simulink library "csc_cgs_coast_guidance_system_lib"  (R2015b)
settings: Solver=ode45  StartTime=0.0  StopTime=10.0  RelTol=1e-3
libraries: util_info_lib x1, util_common_lib x1, csu_arg_aimpoint_roll_guidance_lib x1
settings Model: Creator=Nilesh  LastModifiedBy=Mark Agbayani
settings DataIOCC: SaveFormat=Array
settings DebuggingCC: UnderspecifiedInitializationDetection=Classic  MergeDetectMultiDrivingBlocksExec=none  SolverPrmCheckMsg=warning  StateNameClashWarn=warning
settings HardwareCC: ProdBitPerPointer=32  ProdLargestAtomicFloat=None  ProdIntDivRoundTo=Undefined  ProdEndianess=Unspecified  ProdWordSize=32  ProdHWDeviceType=32-bit Generic
settings GRTTargetCC: GeneratePreprocessorConditionals=Disable all
settings ConfigComp: CovModelRefEnable=Off  CovSFcnEnable=off

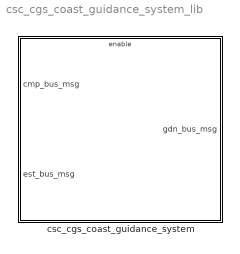
== system csc_cgs_coast_guidance_system_lib ==
  csc_cgs_coast_guidance_system : Subsystem

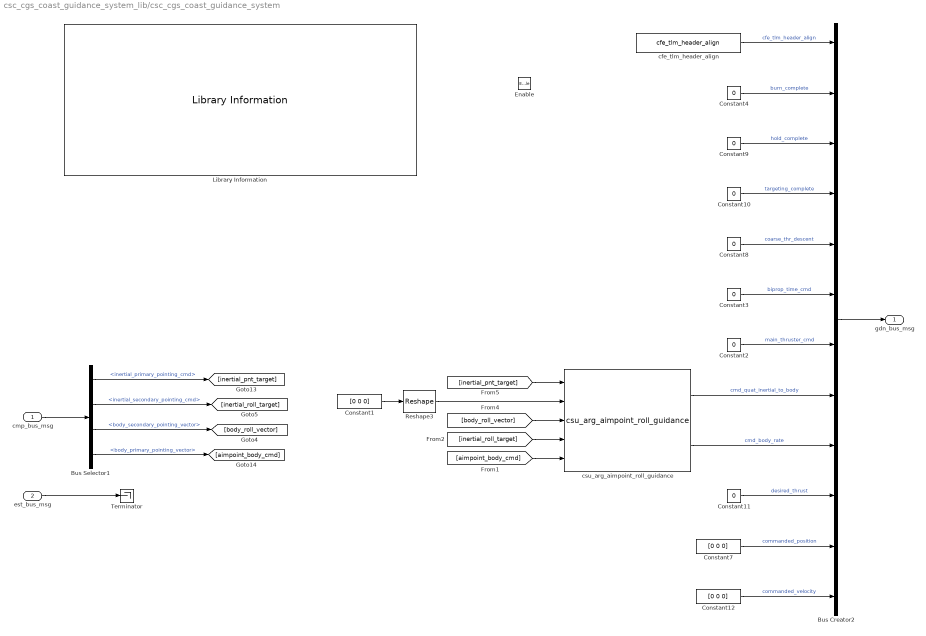
== system csc_cgs_coast_guidance_system_lib/csc_cgs_coast_guidance_system ==
  cmp_bus_msg : Inport
  est_bus_msg : Inport  Port=2
  Enable : EnablePort
  Bus Selector1 : BusSelector  OutputSignals=inertial_primary_pointing_cmd,inertial_secondary_pointing_cmd,body_secondary_pointing_vector,body_primary_pointing_vector
  Bus Creator2 : BusCreator  Inputs=12  OutDataTypeStr=Bus: gdn_bus_msg  NonVirtualBus=on
  Constant1 : Constant  Value=[0 0 0]
  Constant{3..4,8..10} (5 alike) : Constant  Value=0  OutDataTypeStr=uint8
  Constant11 : Constant  Value=0
  Constant12 : Constant  Value=[0 0 0]
  Constant2 : Constant  Value=0
  Constant7 : Constant  Value=[0 0 0]
  Library Information : util_info_lib/Library Information  owner='jkaidy'
  Reshape3 : Reshape  OutputDimensionality=Column vector (2-D)
  Terminator : Terminator
  cfe_tlm_header_align : util_common_lib/cfe_tlm_header_align
  csu_arg_aimpoint_roll_guidance : csu_arg_aimpoint_roll_guidance_lib/csu_arg_aimpoint_roll_guidance
  gdn_bus_msg : Outport  OutDataTypeStr=Bus: gdn_bus_msg
  wires:
  Constant4/1 -> Bus Creator2/2  "burn_complete"
  Constant7/1 -> Bus Creator2/11  "commanded_position"
  Constant12/1 -> Bus Creator2/12  "commanded_velocity"
  Constant3/1 -> Bus Creator2/6  "biprop_time_cmd"
  cfe_tlm_header_align/1 -> Bus Creator2/1  "cfe_tlm_header_align"
  Constant10/1 -> Bus Creator2/4  "targeting_complete"
  Constant9/1 -> Bus Creator2/3  "hold_complete"
  csu_arg_aimpoint_roll_guidance/2 -> Bus Creator2/9  "cmd_body_rate"
  csu_arg_aimpoint_roll_guidance/1 -> Bus Creator2/8  "cmd_quat_inertial_to_body"
  Bus Creator2/1 -> gdn_bus_msg/1
  Constant2/1 -> Bus Creator2/7  "main_thruster_cmd"
  Constant8/1 -> Bus Creator2/5  "coarse_thr_descent"
  Constant11/1 -> Bus Creator2/10  "desired_thrust"
  cmp_bus_msg/1 -> Bus Selector1/1
  Bus Selector1/3 -> [body_roll_vector]  "<body_secondary_pointing_vector>"
  Bus Selector1/2 -> [inertial_roll_target]  "<inertial_secondary_pointing_cmd>"
  Bus Selector1/1 -> [inertial_pnt_target]  "<inertial_primary_pointing_cmd>"
  est_bus_msg/1 -> Terminator/1
  Constant1/1 -> Reshape3/1
  [body_roll_vector] -> csu_arg_aimpoint_roll_guidance/3
  [inertial_roll_target] -> csu_arg_aimpoint_roll_guidance/4
  Reshape3/1 -> csu_arg_aimpoint_roll_guidance/2
  [inertial_pnt_target] -> csu_arg_aimpoint_roll_guidance/1
  Bus Selector1/4 -> [aimpoint_body_cmd]  "<body_primary_pointing_vector>"
  [aimpoint_body_cmd] -> csu_arg_aimpoint_roll_guidance/5
